simulink model "Resp18e_updatedPulse"  (Simulink 7.3)
settings: Solver=ode23  StartTime=0.0  StopTime=20  FixedStep=0.01  MaxStep=0.05  RelTol=1e-6
values from neighbouring files (symbols this model uses):
  alpha_CO2_brain = 2.9/1e3*760/P_stp/K_stp    (= 0.00097047576489)    [initialize_parameters.m]
  alpha_CO2_fat = 0.9/K_stp/P_stp    (= 0.000396292281489)    [initialize_parameters.m]
  alpha_CO2_heart = 2.4/1e3*760/P_stp/K_stp    (= 0.00080315235715)    [initialize_parameters.m]
  alpha_CO2_lean = 4.2/1e3*760/P_stp/K_stp    (= 0.00140551662501)    [initialize_parameters.m]
  alpha_CO2_lungtiss_fast = alpha_CO2_lungtiss_fast./0.1333    [initialize_parameters.m]
  alpha_CO2_muscle = 4.2/1e3*760/P_stp/K_stp    (= 0.00140551662501)    [initialize_parameters.m]
  alpha_CO2_other = 3.0/1e3*760/P_stp/K_stp    (= 0.00100394044644)    [initialize_parameters.m]
  alpha_O2_fat = 5*0.024/K_stp/P_stp    (= 5.28389708651e-05)    [initialize_parameters.m]
  alpha_O2_tissue = 0.024/K_stp/P_stp    (= 1.0567794173e-05)    [initialize_parameters.m]
  BOHRF0 = O2_SHIFT - T_BLOOD_M_37 * (0.024 + BOHRF * 0.0147) - BOHRF1 * 7.4    (= -3.552)    [initialize_parameters.m]
  BOHRF1 = BOHRF * (1 - T_BLOOD_M_37 * 0.0065)    (= 0.48)    [initialize_parameters.m]
  C_a_CO2_i = 20.8e-3    (= 0.0208)    [initialize_parameters.m]    (also in resp18e_ic_norm.mat = 0.0202734801806)
  C_a_O2_i = 8.95e-3    (= 0.00895)    [initialize_parameters.m]    (also in resp18e_ic_norm.mat = 0.00918087581167)
  CAP_O2 = 0.01 * CAP_O2    (= 0.201)    [initialize_parameters.m]
  Cardiac_duty_cycle = 40    [initialize_parameters.m]
  Co_CO2_brain = 401*K_Co_CO2/1e3/K_stp    (= 0.0107345869894)    [initialize_parameters.m]
  Co_CO2_heart = 487*K_Co_CO2/1e3/K_stp    (= 0.0130367677403)    [initialize_parameters.m]
  Co_CO2_lean = 342*K_Co_CO2/1e3/K_stp    (= 0.00915518391618)    [initialize_parameters.m]
  Co_CO2_muscle = 342*K_Co_CO2/1e3/K_stp    (= 0.00915518391618)    [initialize_parameters.m]
  Co_CO2_other = 355*K_Co_CO2/1e3/K_stp    (= 0.00950318798317)    [initialize_parameters.m]
  DH2ODS = DH2ODS + 0.007 * HB_MEQ * (HB_MEQ - 9) / (13.5 * (13.5 - 9))    (= 0.00498709726946)    [initialize_parameters.m]
  F_insp_alv_alvds = F_v_alv_deadspace / F_insp_hivq    (= 0.00299401197605)    [initialize_parameters.m]
  F_insp_alv_hivq = F_v_alv_hivq      / F_insp_hivq    (= 0.997005988024)    [initialize_parameters.m]
  F_insp_alv_lovq = F_v_alv_lovq      / F_insp_lovq    (= 0.5)    [initialize_parameters.m]
  F_insp_alv_midvq = F_v_alv_midvq     / F_insp_lovq    (= 0.5)    [initialize_parameters.m]
  F_insp_hivq = F_v_alv_deadspace + F_v_alv_hivq    (= 0.334)    [initialize_parameters.m]
  F_insp_lovq = F_v_alv_midvq     + F_v_alv_lovq    (= 0.666)    [initialize_parameters.m]
  Fi_CO2_param_est = 0.01    [initialize_parameters.m]
  Fi_error = 1e-6    (= 1e-06)    [initialize_parameters.m]
  Fi_N2_mean = 1-(Fi_O2_mean + Fi_N2O_mean)    (= 0.65)    [initialize_parameters.m]
  Fi_O2_mean = 0.35    [initialize_parameters.m]
  Fi_O2_param_est = 0.01    [initialize_parameters.m]
  Fq_brain = 0.114    [initialize_parameters.m]
  Fq_error = 1e-8    (= 1e-08)    [initialize_parameters.m]
  Fq_fat = 0.103    [initialize_parameters.m]
  Fq_heart = 0.041    [initialize_parameters.m]
  Fq_hepatic = 0.069    [initialize_parameters.m]
  Fq_kidneys = 0.215    [initialize_parameters.m]
  Fq_lean = 0.090    (= 0.09)    [initialize_parameters.m]
  Fq_lungs_anatomicalshunt = 0.01    [initialize_parameters.m]
  Fq_lungs_hivq = (1-Fq_lungs_pulmshunt-Fq_lungs_anatomicalshunt)    *F_v_alv_hivq/(F_v_alv_hivq+F_v_alv_midvq+F_v_alv_lovq)    (= 0.3)    [initialize_parameters.m]
  Fq_lungs_lovq = (1-Fq_lungs_pulmshunt-Fq_lungs_anatomicalshunt)    *F_v_alv_lovq/(F_v_alv_hivq+F_v_alv_midvq+F_v_alv_lovq)    (= 0.3)    [initialize_parameters.m]
  Fq_lungs_midvq = (1-Fq_lungs_pulmshunt-Fq_lungs_anatomicalshunt)    *F_v_alv_midvq/(F_v_alv_hivq+F_v_alv_midvq+F_v_alv_lovq)    (= 0.3)    [initialize_parameters.m]
  Fq_lungs_pulmshunt = 0.09    [initialize_parameters.m]
  Fq_muscle = 0.096    [initialize_parameters.m]
  Fq_pershunt = 0.101    [initialize_parameters.m]
  Fq_portal = 0.171    [initialize_parameters.m]
  FRC = 2.2    [initialize_parameters.m]
  H2OB = H2OVC + 0.938 * (1 - VC_74)    (= 0.840191964286)    [initialize_parameters.m]
  k_CO2_lungtiss_fast_alvds = k_CO2_lungtiss_fast*F_v_alv_deadspace    (= 3.63090772693e-07)    [initialize_parameters.m]
  k_CO2_lungtiss_fast_hivq = k_CO2_lungtiss_fast*F_v_alv_hivq    (= 0.000120909227307)    [initialize_parameters.m]
  k_CO2_lungtiss_fast_lovq = k_CO2_lungtiss_fast*F_v_alv_lovq    (= 0.000120909227307)    [initialize_parameters.m]
  k_CO2_lungtiss_fast_midvq = k_CO2_lungtiss_fast*F_v_alv_midvq    (= 0.000120909227307)    [initialize_parameters.m]
  k_CO2_lungtiss_slow_alvds = k_CO2_lungtiss_slow*F_v_alv_deadspace    (= 4.95123780945e-09)    [initialize_parameters.m]
  k_CO2_lungtiss_slow_hivq = k_CO2_lungtiss_slow*F_v_alv_hivq    (= 1.64876219055e-06)    [initialize_parameters.m]
  k_CO2_lungtiss_slow_lovq = k_CO2_lungtiss_slow*F_v_alv_lovq    (= 1.64876219055e-06)    [initialize_parameters.m]
  k_CO2_lungtiss_slow_midvq = k_CO2_lungtiss_slow*F_v_alv_midvq    (= 1.64876219055e-06)    [initialize_parameters.m]
  K_diff_CO2_hivq = K_diff_CO2*F_v_alv_hivq    (= 0.0014985)    [initialize_parameters.m]
  K_diff_CO2_lovq = K_diff_CO2*F_v_alv_lovq    (= 0.0014985)    [initialize_parameters.m]
  K_diff_CO2_midvq = K_diff_CO2*F_v_alv_midvq    (= 0.0014985)    [initialize_parameters.m]
  K_diff_O2_hivq = K_diff_O2*F_v_alv_hivq    (= 7.326e-05)    [initialize_parameters.m]
  K_diff_O2_lovq = K_diff_O2*F_v_alv_lovq    (= 7.326e-05)    [initialize_parameters.m]
  K_diff_O2_midvq = K_diff_O2*F_v_alv_midvq    (= 7.326e-05)    [initialize_parameters.m]
  K_exp_alv_alvds = 1/1    (= 1)    [initialize_parameters.m]
  K_exp_alv_hivq = 1/1    (= 1)    [initialize_parameters.m]
  K_press = 760/101.325    (= 7.50061682704)    [initialize_parameters.m]
  K_stp = R*(T_stp+273.15)/(P_stp*1000)    (= 22.4135311621)    [initialize_parameters.m]
  Kg_alv = R*(T_alv+273.15)/(P_baro*1000)    (= 25.3668469802)    [initialize_parameters.m]
  LN10 = 2.30258509299405    (= 2.30258509299)    [initialize_parameters.m]
  m_alv_alvds_i = (FRC-V_deadspace_total)/Kg_alv * F_v_alv_deadspace    [initialize_parameters.m]
  m_alv_hivq_i = (FRC-V_deadspace_total)/Kg_alv * F_v_alv_hivq    [initialize_parameters.m]
  m_alv_lovq_i = (FRC-V_deadspace_total)/Kg_alv * F_v_alv_lovq    [initialize_parameters.m]
  m_alv_midvq_i = (FRC-V_deadspace_total)/Kg_alv * F_v_alv_midvq    [initialize_parameters.m]
  m_CO2_alv_alvds_i = F_CO2_i * m_alv_alvds_i    [initialize_parameters.m]
  m_CO2_alv_hivq_i = F_CO2_i * m_alv_hivq_i    [initialize_parameters.m]
  m_CO2_alv_lovq_i = F_CO2_i * m_alv_lovq_i    [initialize_parameters.m]
  m_CO2_alv_midvq_i = F_CO2_i * m_alv_midvq_i    [initialize_parameters.m]
  m_CO2_brain_b_i = C_a_CO2_i*Vb_brain    (= 0.002184)    [initialize_parameters.m]
  m_CO2_brain_t_i = (Co_CO2_brain  + alpha_CO2_brain *P_v_CO2_i)* Vt_brain    (= 0.0171268217946)    [initialize_parameters.m]
  m_CO2_common_b_i = C_a_CO2_i*Vb_common    (= 0.0170421333333)    [initialize_parameters.m]
  m_CO2_ds0_i = F_CO2_i*m_ds0_i    (= 0.000985538329597)    [initialize_parameters.m]
  m_CO2_ds_large_i = F_CO2_i * m_deadspace_large_1    [initialize_parameters.m]
  m_CO2_ds_med_hivq1_i = F_CO2_i * m_deadspace_med_hivq_1    [initialize_parameters.m]
  m_CO2_ds_med_hivq2_i = F_CO2_i * m_deadspace_med_hivq_2    [initialize_parameters.m]
  m_CO2_ds_med_lovq1_i = F_CO2_i * m_deadspace_med_lovq_1    [initialize_parameters.m]
  m_CO2_ds_med_lovq2_i = F_CO2_i * m_deadspace_med_lovq_2    [initialize_parameters.m]
  m_CO2_ds_small_alvds_i = F_CO2_i * m_deadspace_small_alvdeadspace    [initialize_parameters.m]
  m_CO2_ds_small_hivq_i = F_CO2_i * m_deadspace_small_hivq    [initialize_parameters.m]
  m_CO2_ds_small_lovq_i = F_CO2_i * m_deadspace_small_lovq    [initialize_parameters.m]
  m_CO2_ds_small_midvq_i = F_CO2_i * m_deadspace_small_midvq    [initialize_parameters.m]
  m_CO2_fat_b_i = C_a_CO2_i*Vb_fat    (= 0.0116896)    [initialize_parameters.m]
  m_CO2_fat_t_i = P_a_CO2_i*alpha_CO2_fat*Vt_fat    (= 0.0302752719501)    [initialize_parameters.m]
  m_CO2_heart_b_i = C_a_CO2_i*Vb_heart    (= 0.000832)    [initialize_parameters.m]
  m_CO2_heart_t_i = (Co_CO2_heart  + alpha_CO2_heart *P_v_CO2_i)* Vt_heart    (= 0.00402544335149)    [initialize_parameters.m]
  m_CO2_hepatic_b_i = C_a_CO2_i*Vb_hepatic    (= 0.0019136)    [initialize_parameters.m]
  m_CO2_kidneys_b_i = C_a_CO2_i*Vb_kidneys    (= 0.0012064)    [initialize_parameters.m]
  m_CO2_kidneys_t_i = (Co_CO2_other  + alpha_CO2_other *P_v_CO2_i)* Vt_kidneys    (= 0.0045902552907)    [initialize_parameters.m]
  m_CO2_lean_b_i = C_a_CO2_i*Vb_lean    (= 0.0191984)    [initialize_parameters.m]
  m_CO2_lean_t_i = (Co_CO2_lean   + alpha_CO2_lean  *P_v_CO2_i)* Vt_lean    (= 0.0884995401953)    [initialize_parameters.m]
  m_CO2_liver_t_i = (Co_CO2_other  + alpha_CO2_other *P_v_CO2_i)* Vt_liver    (= 0.0187019339777)    [initialize_parameters.m]
  m_CO2_lungtiss_fast_alvds_i = F_CO2_i*(P_baro-P_A_H2O)*V_lungtiss_alvds *alpha_CO2_lungtiss_fast(2)    [initialize_parameters.m]
  m_CO2_lungtiss_fast_hivq_i = F_CO2_i*(P_baro-P_A_H2O)*V_lungtiss_hivq  *alpha_CO2_lungtiss_fast(2)    [initialize_parameters.m]
  m_CO2_lungtiss_fast_lovq_i = F_CO2_i*(P_baro-P_A_H2O)*V_lungtiss_lovq  *alpha_CO2_lungtiss_fast(2)    [initialize_parameters.m]
  m_CO2_lungtiss_fast_midvq_i = F_CO2_i*(P_baro-P_A_H2O)*V_lungtiss_midvq *alpha_CO2_lungtiss_fast(2)    [initialize_parameters.m]
  m_CO2_lungtiss_slow_alvds_i = F_CO2_i*(P_baro-P_A_H2O)*V_lungtiss_alvds*alpha_CO2_lungtiss_slow    [initialize_parameters.m]
  m_CO2_lungtiss_slow_hivq_i = F_CO2_i*(P_baro-P_A_H2O)*V_lungtiss_hivq *alpha_CO2_lungtiss_slow    [initialize_parameters.m]
  m_CO2_lungtiss_slow_lovq_i = F_CO2_i*(P_baro-P_A_H2O)*V_lungtiss_lovq *alpha_CO2_lungtiss_slow    [initialize_parameters.m]
  m_CO2_lungtiss_slow_midvq_i = F_CO2_i*(P_baro-P_A_H2O)*V_lungtiss_midvq*alpha_CO2_lungtiss_slow    [initialize_parameters.m]
  m_CO2_LV_b_i = C_a_CO2_i*Vb_LV    (= 0.00391733333333)    [initialize_parameters.m]
  m_CO2_muscle_b_i = C_a_CO2_i*Vb_muscle    (= 0.0201344)    [initialize_parameters.m]
  m_CO2_muscle_t_i = (Co_CO2_muscle + alpha_CO2_muscle*P_v_CO2_i)* Vt_muscle    (= 0.363660431061)    [initialize_parameters.m]
  m_CO2_pershunt_b_i = C_a_CO2_i*Vb_pershunt    (= 0.0027248)    [initialize_parameters.m]
  m_CO2_portal_b_i = C_a_CO2_i*Vb_portal    (= 0.0210912)    [initialize_parameters.m]
  m_CO2_portal_t_i = (Co_CO2_other  + alpha_CO2_other *P_v_CO2_i)* Vt_portal    (= 0.0164739329706)    [initialize_parameters.m]
  m_CO2_pulmcap_b_hivq_i = C_a_CO2_i*Vb_pulmcap_hivq    (= 0.000630933333333)    [initialize_parameters.m]
  m_CO2_pulmcap_b_lovq_i = C_a_CO2_i*Vb_pulmcap_lovq    (= 0.000630933333333)    [initialize_parameters.m]
  m_CO2_pulmcap_b_midvq_i = C_a_CO2_i*Vb_pulmcap_midvq    (= 0.000630933333333)    [initialize_parameters.m]
  m_CO2_pulmcap_b_pulmshunt_i = C_a_CO2_i*Vb_pulmcap_pulmshunt    (= 0.0001872)    [initialize_parameters.m]
  m_CO2_RV_b_i = C_v_CO2_i*Vb_RV    (= 0.004181)    [initialize_parameters.m]
  m_N2_alv_alvds_i = Fi_N2_mean * (m_alv_alvds_i - m_CO2_alv_alvds_i)    [initialize_parameters.m]
  ... (+122 more)
undefined symbols (not defined in the file or in its folder): AH2OVC, AHCO3B, DHCO3BDS, litres, mole
libraries: simulink x28
(part 2 of 8)

== system Resp18e_updatedPulse/Patient/Pulm cap Hi V/Q ==
  note: This block calculates:
      | 1. Alveolar partial pressures of CO2 & O2
      | 2. CO2 uptake by lung tissues
      | 3. CO2 uptake by pulmonary capillaries
      | 4. O2 uptake by pulmonary capillaries
  note: Variables:
      | CA_CO2: alveolar CO2 fraction (pu)
      | CA_O2: alveolar O2 fraction (pu)
      | P_baro: barometric pressure (kPa)
      | P_alv: gauge pressure in alveolar compartment (kPa)
      | P_H2O_alv: partial press of H2O vapour in alveolar compartment (kPa)
      | C_v_CO2: mixed venous CO2 concentration (moles/l)
      | C_v_O2: mixed venous O2 concentration (moles/l)
      | Qpdot: pulmonary blood flow (l/sec)
      | mdot_CO2_tiss_cap: flux of CO2 from alv to tissues + pulm capillaries (mole/sec)
      | mdot_O2_tiss_cap: flux of O2 from alv to tissues + pulm capillaries (mole/sec)
      | Cec_CO2 CO2 conc at end of pulm capillaries
      | Cec_O2 O2 conc at end of pulm capillaries
      | CaCO2: arterial CO2 concentration (moles/l)
      | CaO2: arterial O2 concentration (moles/l)
  FA_gases : Inport  PortDimensions=2  OutDataType=sfix(16)  OutScaling=2^0
  C_v_gases : Inport  Port=2  PortDimensions=2  OutDataType=sfix(16)  OutScaling=2^0
  CO2 O2 : Mux  Inputs=2
  Demux : Demux  Outputs=2
  Lung tissue : Subsystem  Description=Calculates quantity of CO2 stored in two lung tissue compartments (fast & slow)
  Net inflow CO4 : Sum  OutDataType=sfix(16)  OutScaling=2^0  SaturateOnIntegerOverflow=on  InputSameDT=on  OutDataTypeStr=Inherit: Same as first input
  P3 : Product  Inputs=**  OutDataType=sfix(16)  OutScaling=2^0  SaturateOnIntegerOverflow=on  RndMeth=Zero  InputSameDT=on  OutDataTypeStr=Inherit: Same as first input
  P4 : Product  Inputs=**  OutDataType=sfix(16)  OutScaling=2^0  SaturateOnIntegerOverflow=on  RndMeth=Zero  InputSameDT=on  OutDataTypeStr=Inherit: Same as first input
  Pulm capillaries : Subsystem
  To Workspace16 : ToWorkspace  VariableName=mdot_CO2_a_A_hivq  SampleTime=t_sample  SaveFormat=Array
  To Workspace8 : ToWorkspace  VariableName=P_A_CO2_hivq  SampleTime=t_sample  SaveFormat=Array
  To Workspace9 : ToWorkspace  VariableName=P_A_O2_hivq  SampleTime=t_sample  SaveFormat=Array
  sum3 : Sum  Inputs=++-  OutDataType=sfix(16)  OutScaling=2^0  SaturateOnIntegerOverflow=on  InputSameDT=on  OutDataTypeStr=Inherit: Same as first input
  mdot_gases : Outport  OutDataType=sfix(16)  OutScaling=2^0
  C_gases : Outport  Port=2  OutDataType=sfix(16)  OutScaling=2^0
  tag scope: mdot_CO2_a_A_hivq=global, mdot_O2_a_A_hivq=global
  wires:
  Lung tissue/1(mdot_CO2_tissue) -> Net inflow CO4/1
  sum3/1 -> P3/2, P4/2
  P3/1 -> Pulm capillaries/1(PA_CO2), Lung tissue/1(PA_CO2), To Workspace8/1  "PA_CO2"
  Demux/2 -> P4/1
  P4/1 -> Pulm capillaries/2(PA_O2), To Workspace9/1  "PA_O2"
  Demux/1 -> P3/1
  Net inflow CO4/1 -> CO2 O2/1
  CO2 O2/1 -> mdot_gases/1
  [P_alv] -> sum3/2
  FA_gases/1 -> Demux/1
  Pulm capillaries/1(mdot_CO2_A_a) -> Net inflow CO4/2, To Workspace16/1, [mdot_CO2_a_A_hivq]
  [P_A_H2O] -> sum3/3
  [P_baro] -> sum3/1
  C_v_gases/1 -> Pulm capillaries/3(C_v_gases)
  Pulm capillaries/3(Cec_gases) -> C_gases/1
  Pulm capillaries/2(mdot_O2_A_a) -> CO2 O2/2, [mdot_O2_a_A_hivq]

== system Resp18e_updatedPulse/Patient/Pulm cap Lo V/Q ==
  note: This block calculates:
      | 1. Alveolar partial pressures of CO2 & O2
      | 2. CO2 uptake by lung tissues
      | 3. CO2 uptake by pulmonary capillaries
      | 4. O2 uptake by pulmonary capillaries
  note: Variables:
      | CA_CO2: alveolar CO2 fraction (pu)
      | CA_O2: alveolar O2 fraction (pu)
      | P_baro: barometric pressure (kPa)
      | P_alv: gauge pressure in alveolar compartment (kPa)
      | P_H2O_alv: partial press of H2O vapour in alveolar compartment (kPa)
      | C_v_CO2: mixed venous CO2 concentration (moles/l)
      | C_v_O2: mixed venous O2 concentration (moles/l)
      | Qpdot: pulmonary blood flow (l/sec)
      | mdot_CO2_tiss_cap: flux of CO2 from alv to tissues + pulm capillaries (mole/sec)
      | mdot_O2_tiss_cap: flux of O2 from alv to tissues + pulm capillaries (mole/sec)
      | Cec_CO2 CO2 conc at end of pulm capillaries
      | Cec_O2 O2 conc at end of pulm capillaries
      | CaCO2: arterial CO2 concentration (moles/l)
      | CaO2: arterial O2 concentration (moles/l)
  FA_gases : Inport  PortDimensions=2  OutDataType=sfix(16)  OutScaling=2^0
  C_v_gases : Inport  Port=2  PortDimensions=2  OutDataType=sfix(16)  OutScaling=2^0
  CO2 O2 : Mux  Inputs=2
  Demux : Demux  Outputs=2
  Lung tissue : Subsystem  Description=Calculates quantity of CO2 stored in two lung tissue compartments (fast & slow)
  Net inflow CO4 : Sum  OutDataType=sfix(16)  OutScaling=2^0  SaturateOnIntegerOverflow=on  InputSameDT=on  OutDataTypeStr=Inherit: Same as first input
  P3 : Product  Inputs=**  OutDataType=sfix(16)  OutScaling=2^0  SaturateOnIntegerOverflow=on  RndMeth=Zero  InputSameDT=on  OutDataTypeStr=Inherit: Same as first input
  P4 : Product  Inputs=**  OutDataType=sfix(16)  OutScaling=2^0  SaturateOnIntegerOverflow=on  RndMeth=Zero  InputSameDT=on  OutDataTypeStr=Inherit: Same as first input
  Pulm capillaries : Subsystem
  To Workspace16 : ToWorkspace  VariableName=mdot_CO2_a_A_lovq  SampleTime=t_sample  SaveFormat=Array
  To Workspace8 : ToWorkspace  VariableName=P_A_CO2_lovq  SampleTime=t_sample  SaveFormat=Array
  To Workspace9 : ToWorkspace  VariableName=P_A_O2_lovq  SampleTime=t_sample  SaveFormat=Array
  sum3 : Sum  Inputs=++-  OutDataType=sfix(16)  OutScaling=2^0  SaturateOnIntegerOverflow=on  InputSameDT=on  OutDataTypeStr=Inherit: Same as first input
  mdot_gases : Outport  OutDataType=sfix(16)  OutScaling=2^0
  C_gases : Outport  Port=2  OutDataType=sfix(16)  OutScaling=2^0
  tag scope: mdot_CO2_a_A_lovq=global, mdot_O2_a_A_lovq=global
  wires:
  Lung tissue/1(mdot_CO2_tissue) -> Net inflow CO4/1
  sum3/1 -> P3/2, P4/2
  P3/1 -> Pulm capillaries/1(PA_CO2), Lung tissue/1(PA_CO2), To Workspace8/1  "PA_CO2"
  Demux/2 -> P4/1
  P4/1 -> Pulm capillaries/2(PA_O2), To Workspace9/1  "PA_O2"
  Demux/1 -> P3/1
  Net inflow CO4/1 -> CO2 O2/1
  CO2 O2/1 -> mdot_gases/1
  [P_alv] -> sum3/2
  FA_gases/1 -> Demux/1
  Pulm capillaries/1(mdot_CO2_A_a) -> Net inflow CO4/2, To Workspace16/1, [mdot_CO2_a_A_lovq]
  [P_A_H2O] -> sum3/3
  [P_baro] -> sum3/1
  C_v_gases/1 -> Pulm capillaries/3(C_v_gases)
  Pulm capillaries/3(Cec_gases) -> C_gases/1
  Pulm capillaries/2(mdot_O2_A_a) -> CO2 O2/2, [mdot_O2_a_A_lovq]

== system Resp18e_updatedPulse/Patient/Pulm cap Mid V/Q ==
  note: Variables:
      | CA_CO2: alveolar CO2 fraction (pu)
      | CA_O2: alveolar O2 fraction (pu)
      | P_baro: barometric pressure (kPa)
      | P_alv: gauge pressure in alveolar compartment (kPa)
      | P_H2O_alv: partial press of H2O vapour in alveolar compartment (kPa)
      | C_v_CO2: mixed venous CO2 concentration (moles/l)
      | C_v_O2: mixed venous O2 concentration (moles/l)
      | Qpdot: pulmonary blood flow (l/sec)
      | mdot_CO2_tiss_cap: flux of CO2 from alv to tissues + pulm capillaries (mole/sec)
      | mdot_O2_tiss_cap: flux of O2 from alv to tissues + pulm capillaries (mole/sec)
      | Cec_CO2 CO2 conc at end of pulm capillaries
      | Cec_O2 O2 conc at end of pulm capillaries
      | CaCO2: arterial CO2 concentration (moles/l)
      | CaO2: arterial O2 concentration (moles/l)
  note: This block calculates:
      | 1. Alveolar partial pressures of CO2 & O2
      | 2. CO2 uptake by lung tissues
      | 3. CO2 uptake by pulmonary capillaries
      | 4. O2 uptake by pulmonary capillaries
  FA_gases : Inport  PortDimensions=2  OutDataType=sfix(16)  OutScaling=2^0
  C_v_gases : Inport  Port=2  PortDimensions=2  OutDataType=sfix(16)  OutScaling=2^0
  CO2 O2 : Mux  Inputs=2
  Demux : Demux  Outputs=2
  Lung tissue : Subsystem  Description=Calculates quantity of CO2 stored in two lung tissue compartments (fast & slow)
  Net inflow CO4 : Sum  OutDataType=sfix(16)  OutScaling=2^0  SaturateOnIntegerOverflow=on  InputSameDT=on  OutDataTypeStr=Inherit: Same as first input
  P3 : Product  Inputs=**  OutDataType=sfix(16)  OutScaling=2^0  SaturateOnIntegerOverflow=on  RndMeth=Zero  InputSameDT=on  OutDataTypeStr=Inherit: Same as first input
  P4 : Product  Inputs=**  OutDataType=sfix(16)  OutScaling=2^0  SaturateOnIntegerOverflow=on  RndMeth=Zero  InputSameDT=on  OutDataTypeStr=Inherit: Same as first input
  Pulm capillaries : Subsystem
  To Workspace16 : ToWorkspace  VariableName=mdot_CO2_a_A_midvq  SampleTime=t_sample  SaveFormat=Array
  To Workspace17 : ToWorkspace  VariableName=mdot_CO2_A_midvq  SampleTime=t_sample  SaveFormat=Array
  To Workspace8 : ToWorkspace  VariableName=P_A_CO2_midvq  SampleTime=t_sample  SaveFormat=Array
  To Workspace9 : ToWorkspace  VariableName=P_A_O2_midvq  SampleTime=t_sample  SaveFormat=Array
  sum3 : Sum  Inputs=++-  OutDataType=sfix(16)  OutScaling=2^0  SaturateOnIntegerOverflow=on  InputSameDT=on  OutDataTypeStr=Inherit: Same as first input
  mdot_gases : Outport  OutDataType=sfix(16)  OutScaling=2^0
  C_gases : Outport  Port=2  OutDataType=sfix(16)  OutScaling=2^0
  tag scope: mdot_CO2_a_A_midvq=global, mdot_O2_a_A_midvq=global
  wires:
  Pulm capillaries/3(Cec_gases) -> C_gases/1
  C_v_gases/1 -> Pulm capillaries/3(C_v_gases)
  [P_baro] -> sum3/1
  [P_A_H2O] -> sum3/3
  Pulm capillaries/1(mdot_CO2_A_a) -> Net inflow CO4/2, To Workspace16/1, [mdot_CO2_a_A_midvq]
  FA_gases/1 -> Demux/1
  [P_alv] -> sum3/2
  CO2 O2/1 -> mdot_gases/1
  Demux/1 -> P3/1
  P4/1 -> To Workspace9/1, Pulm capillaries/2(PA_O2)  "PA_O2"
  Demux/2 -> P4/1
  P3/1 -> To Workspace8/1, Lung tissue/1(PA_CO2), Pulm capillaries/1(PA_CO2)  "PA_CO2"
  sum3/1 -> P4/2, P3/2
  Lung tissue/1(mdot_CO2_tissue) -> Net inflow CO4/1
  Net inflow CO4/1 -> CO2 O2/1, To Workspace17/1
  Pulm capillaries/2(mdot_O2_A_a) -> CO2 O2/2, [mdot_O2_a_A_midvq]

== system Resp18e_updatedPulse/Patient/Pulm cap pulm shunt ==
  note: Pulmonary capillary shunt
  note: This block calculates mixing and effective delay in pulmonary capillary compartment that is not exposed to alveolar gas
      | Note that the time constant of this 1st order loop should be approx independent of V_b_pulmcap_pulmshunt if
      | V_b_pulmcap_pulmshunt is approx proportional to Fq_lung_pulmshunt
  C_v_gases : Inport  PortDimensions=2  OutDataType=sfix(16)  OutScaling=2^0
  CO2_cap : Integrator  InitialCondition=m_CO2_pulmcap_b_pulmshunt_i
  C_CO2 body : Gain  Gain=1/Vb_pulmcap_pulmshunt  ParameterDataType=sfix(16)  ParameterScaling=2^0  OutDataType=sfix(16)  OutScaling=2^0  SaturateOnIntegerOverflow=on  OutDataTypeStr=Inherit: Same as input  ParamDataTypeStr=Inherit: Same as input
  C_O2 body : Gain  Gain=1/Vb_pulmcap_pulmshunt  ParameterDataType=sfix(16)  ParameterScaling=2^0  OutDataType=sfix(16)  OutScaling=2^0  SaturateOnIntegerOverflow=on  OutDataTypeStr=Inherit: Same as input  ParamDataTypeStr=Inherit: Same as input
  Demux2 : Demux  Outputs=2
  Mux1 : Mux  Inputs=2
  Net inflow CO5 : Sum  Inputs=+-  OutDataType=sfix(16)  OutScaling=2^0  SaturateOnIntegerOverflow=on  InputSameDT=on  OutDataTypeStr=Inherit: Same as first input
  Net inflow CO6 : Sum  Inputs=+-  OutDataType=sfix(16)  OutScaling=2^0  SaturateOnIntegerOverflow=on  InputSameDT=on  OutDataTypeStr=Inherit: Same as first input
  O2_cap : Integrator  InitialCondition=m_O2_pulmcap_b_pulmshunt_i
  P11 : Product  Inputs=**  OutDataType=sfix(16)  OutScaling=2^0  SaturateOnIntegerOverflow=on  RndMeth=Zero  InputSameDT=on  OutDataTypeStr=Inherit: Same as first input
  P8 : Product  Inputs=**  OutDataType=sfix(16)  OutScaling=2^0  SaturateOnIntegerOverflow=on  RndMeth=Zero  InputSameDT=on  OutDataTypeStr=Inherit: Same as first input
  P9 : Product  Inputs=**  OutDataType=sfix(16)  OutScaling=2^0  SaturateOnIntegerOverflow=on  RndMeth=Zero  InputSameDT=on  OutDataTypeStr=Inherit: Same as first input
  Cec_gases : Outport  OutDataType=sfix(16)  OutScaling=2^0
  wires:
  CO2_cap/1 -> C_CO2 body/1
  O2_cap/1 -> C_O2 body/1
  Net inflow CO5/1 -> P8/1
  Demux2/1 -> Net inflow CO5/1
  Demux2/2 -> Net inflow CO6/1
  Net inflow CO6/1 -> P9/2
  P8/1 -> CO2_cap/1
  P9/1 -> O2_cap/1
  C_CO2 body/1 -> Net inflow CO5/2, Mux1/1
  C_O2 body/1 -> Net inflow CO6/2, Mux1/2
  Mux1/1 -> Cec_gases/1
  [Fq_lungs_pulmshunt] -> P11/2
  P11/1 -> P8/2, P9/1
  C_v_gases/1 -> Demux2/1
  [Qpdot] -> P11/1

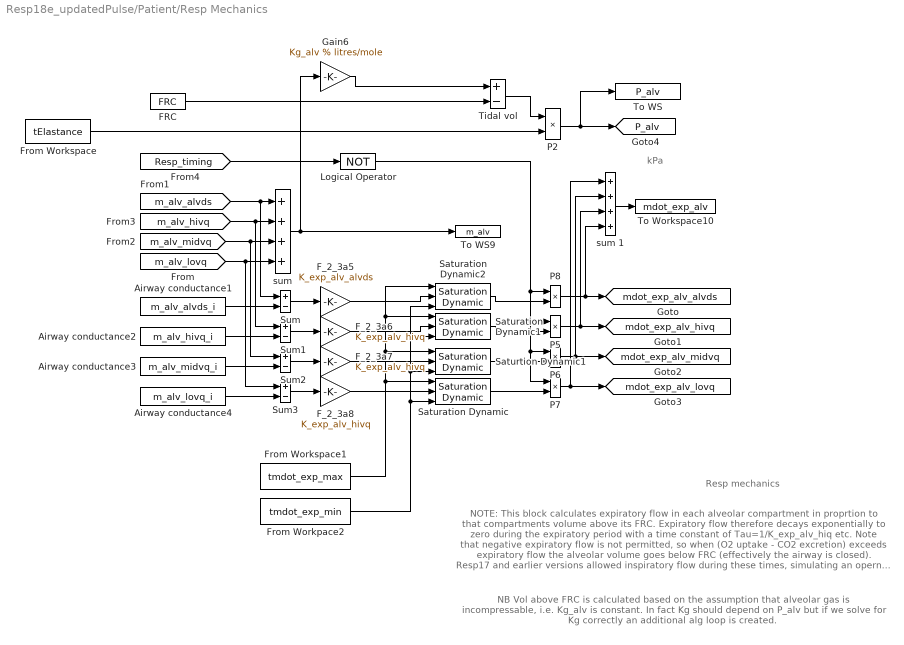
== system Resp18e_updatedPulse/Patient/Resp Mechanics ==
  note: Resp mechanics
  note: NB Vol above FRC is calculated based on the assumption that alveolar gas is incompressable, i.e. Kg_alv
      | is constant. In fact Kg should depend on P_alv but if we solve for Kg correctly an additional alg loop is created.
  note: kPa
  note: NOTE: This block calculates expiratory flow in each alveolar compartment in proprtion to that
      | compartments volume above its FRC. Expiratory flow therefore decays exponentially to
      | zero during the expiratory period with a time constant of Tau=1/K_exp_alv_hiq etc.
      | Note that negative expiratory flow is not permitted, so when (O2 uptake - CO2 excretion)
      | exceeds expiratory flow the alveolar volume goes below FRC (effectively the airway is closed).
      | Resp17 and earlier versions allowed inspiratory flow during these times, simulating an opern airway.
  Airway conductance1 : Constant  Value=m_alv_alvds_i  OutDataType=sfix(16)  OutScaling=2^0
  Airway conductance2 : Constant  Value=m_alv_hivq_i  OutDataType=sfix(16)  OutScaling=2^0
  Airway conductance3 : Constant  Value=m_alv_midvq_i  OutDataType=sfix(16)  OutScaling=2^0
  Airway conductance4 : Constant  Value=m_alv_lovq_i  OutDataType=sfix(16)  OutScaling=2^0
  FRC : Constant  Value=FRC  OutDataType=sfix(16)  OutScaling=2^0
  F_2_3a5 : Gain  Gain=K_exp_alv_alvds  ParameterDataType=sfix(16)  ParameterScaling=2^0  OutDataType=sfix(16)  OutScaling=2^0  SaturateOnIntegerOverflow=on  OutDataTypeStr=Inherit: Same as input  ParamDataTypeStr=Inherit: Same as input
  F_2_3a6 : Gain  Gain=K_exp_alv_hivq  ParameterDataType=sfix(16)  ParameterScaling=2^0  OutDataType=sfix(16)  OutScaling=2^0  SaturateOnIntegerOverflow=on  OutDataTypeStr=Inherit: Same as input  ParamDataTypeStr=Inherit: Same as input
  F_2_3a7 : Gain  Gain=K_exp_alv_hivq  ParameterDataType=sfix(16)  ParameterScaling=2^0  OutDataType=sfix(16)  OutScaling=2^0  SaturateOnIntegerOverflow=on  OutDataTypeStr=Inherit: Same as input  ParamDataTypeStr=Inherit: Same as input
  F_2_3a8 : Gain  Gain=K_exp_alv_hivq  ParameterDataType=sfix(16)  ParameterScaling=2^0  OutDataType=sfix(16)  OutScaling=2^0  SaturateOnIntegerOverflow=on  OutDataTypeStr=Inherit: Same as input  ParamDataTypeStr=Inherit: Same as input
  From Workpace2 : FromWorkspace  VariableName=tmdot_exp_min  SampleTime=0  Interpolate=off  OutputAfterFinalValue=Holding final value
  From Workspace : FromWorkspace  VariableName=tElastance  SampleTime=0  Interpolate=off  OutputAfterFinalValue=Holding final value
  From Workspace1 : FromWorkspace  VariableName=tmdot_exp_max  SampleTime=0  Interpolate=off  OutputAfterFinalValue=Holding final value
  Gain6 : Gain  Gain=Kg_alv % litres/mole  ParameterDataType=sfix(16)  ParameterScaling=2^0  OutDataType=sfix(16)  OutScaling=2^0  SaturateOnIntegerOverflow=on  OutDataTypeStr=Inherit: Same as input  ParamDataTypeStr=Inherit: Same as input
  Logical Operator : Logic  Operator=NOT
  P{2,5..8} (5 alike) : Product  OutDataType=sfix(16)  OutScaling=2^0  SaturateOnIntegerOverflow=on  RndMeth=Zero  InputSameDT=on  OutDataTypeStr=Inherit: Same as first input
  Saturation Dynamic : simulink/Discontinuities/Saturation Dynamic  SystemSampleTime=-1  OutMin=[]  OutMax=[]  OutDataTypeStr=Inherit: Same as second input  OutDataType=fixdt(1, 16)  OutScaling=2^-10  DoSatur=off
  Saturation Dynamic1 : simulink/Discontinuities/Saturation Dynamic  SystemSampleTime=-1  OutMin=[]  OutMax=[]  OutDataTypeStr=Inherit: Same as second input  OutDataType=fixdt(1, 16)  OutScaling=2^-10  DoSatur=off
  Saturation Dynamic2 : simulink/Discontinuities/Saturation Dynamic  SystemSampleTime=-1  OutMin=[]  OutMax=[]  OutDataTypeStr=Inherit: Same as second input  OutDataType=fixdt(1, 16)  OutScaling=2^-10  DoSatur=off
  Saturtion Dynamic1 : simulink/Discontinuities/Saturation Dynamic  SystemSampleTime=-1  OutMin=[]  OutMax=[]  OutDataTypeStr=Inherit: Same as second input  OutDataType=fixdt(1, 16)  OutScaling=2^-10  DoSatur=off
  Sum{,1..3} (4 alike) : Sum  Inputs=+-  OutDataType=sfix(16)  OutScaling=2^0  SaturateOnIntegerOverflow=on  InputSameDT=on  OutDataTypeStr=Inherit: Same as first input
  Tidal vol : Sum  Inputs=+-  OutDataType=sfix(16)  OutScaling=2^0  SaturateOnIntegerOverflow=on  InputSameDT=on  OutDataTypeStr=Inherit: Same as first input
  To WS : ToWorkspace  VariableName=P_alv  SampleTime=t_sample  SaveFormat=Array
  To WS9 : ToWorkspace  VariableName=m_alv  SampleTime=t_sample  SaveFormat=Array
  To Workspace10 : ToWorkspace  VariableName=mdot_exp_alv  SampleTime=t_sample  SaveFormat=Array
  "sum " : Sum  Inputs=++++  OutDataType=sfix(16)  OutScaling=2^0  SaturateOnIntegerOverflow=on  InputSameDT=on  OutDataTypeStr=Inherit: Same as first input
  sum 1 : Sum  Inputs=++++  OutDataType=sfix(16)  OutScaling=2^0  SaturateOnIntegerOverflow=on  InputSameDT=on  OutDataTypeStr=Inherit: Same as first input
  tag scope: P_alv=global, mdot_exp_alv_alvds=global, mdot_exp_alv_hivq=global, mdot_exp_alv_lovq=global, mdot_exp_alv_midvq=global
  wires:
  [m_alv_alvds] -> "sum "/1, Sum/1
  Airway conductance1/1 -> Sum/2
  Airway conductance2/1 -> Sum1/2
  Airway conductance3/1 -> Sum2/2
  Airway conductance4/1 -> Sum3/2
  [m_alv_hivq] -> "sum "/2, Sum1/1
  [m_alv_midvq] -> "sum "/3, Sum2/1
  [m_alv_lovq] -> "sum "/4, Sum3/1
  Sum/1 -> F_2_3a5/1
  F_2_3a5/1 -> Saturation Dynamic2/2
  F_2_3a6/1 -> Saturation Dynamic1/2
  Sum1/1 -> F_2_3a6/1
  F_2_3a7/1 -> Saturtion Dynamic1/2
  F_2_3a8/1 -> Saturation Dynamic/2
  Sum2/1 -> F_2_3a7/1
  Sum3/1 -> F_2_3a8/1
  Saturation Dynamic2/1 -> P8/2
  Saturation Dynamic1/1 -> P5/2
  Saturation Dynamic/1 -> P7/2
  Saturtion Dynamic1/1 -> P6/2
  Logical Operator/1 -> P8/1, P5/1, P6/1, P7/1
  FRC/1 -> Tidal vol/2
  Tidal vol/1 -> P2/1
  Gain6/1 -> Tidal vol/1
  From Workspace/1 -> P2/2
  "sum "/1 -> To WS9/1, Gain6/1
  P2/1 -> To WS/1, [P_alv]
  sum 1/1 -> To Workspace10/1
  P8/1 -> [mdot_exp_alv_alvds], sum 1/4
  P5/1 -> [mdot_exp_alv_hivq], sum 1/3
  P6/1 -> [mdot_exp_alv_midvq], sum 1/2
  P7/1 -> [mdot_exp_alv_lovq], sum 1/1
  [Resp_timing] -> Logical Operator/1
  From Workspace1/1 -> Saturation Dynamic2/1, Saturation Dynamic1/1, Saturtion Dynamic1/1, Saturation Dynamic/1
  From Workpace2/1 -> Saturation Dynamic2/3, Saturation Dynamic1/3, Saturtion Dynamic1/3, Saturation Dynamic/3

== system Resp18e_updatedPulse/Patient/Resp18e Info ==
  note: Initial conditions and parameters taken from work space
  note: Grodins 5 contains an arterial conmpartment, and Simulink variable delays.
  note: Uses Grodins tissue dissociation curves
  note: Grodins5a has Pulm capillary blood compartment
  note: Grodins6 has body tissue compartment
  note: Grodins 7 closes the loop - feeds body venous blood back to mixed venous input
  note: Grodins8 has a 1st order component simulating mixing in heart & aorta
  note: Grodins10 has multiple body compartments
  note: Grodins11 has xport delays in pulmonary artery & vein, & shunt around pulm capillaries
  note: Grodins12 has more than 2 body compartments
  note: Pulm vein + pulm art delays lumped into one
  note: Grodins13 has multiple body compartments based on Mapleson's models
  note: Grodins14 for trying out rebreathing & sinusoid measurements
  note: Grodins15 has high pass filter in CO2 delivery signal to try to cancel the lung ventilation pole
  note: Resp15 has linear tissue CO2 dissociation curves with values from Fahri & Rahn 1960
  note: Resp 16 uses Olszowka's diss curves
  note: Resp 17 has four lung compartments each with their own perfusion. Pure shunt remains
  note: All lung parameters (tissue vol, ventilation diffusion coeffts) etc are set proportional to compartment volumes
  note: Resp18 created to change expiratory flow calculations so that each alv compartment has exp flow in proportion
      | to its volume Exp flow calculated for each alv compartment separately using a time constant parameter
  note: Resp18a has additional integrators for measuring expired CO2 per breath
      | and code for delivering inspired m_CO2 equal to expired m_CO2
  note: Resp18b has code for delivering sinusoidal inspired CO2
  note: Resp18c: identical to Resp18b but has arterial O2 saturation monitoring
  note: Resp18d has pulse generator to control rebreathing so rebreathing measurements can be repeated
  note: Resp18e can deliver CO2 & O2 pulses and decreases inspired N2 accordingly. Developed
      | to generate 'measured' data from which alveolar vol, dead space, mixed venous CO2
      | & O2 and PBF parameter estimation can be done.

== system Resp18e_updatedPulse/Patient/Airways + alveoli/Alv compartment alvds ==
  note: molar conc
      | per unit
  note: +ve out of alv
  Insp flow in : Inport  PortDimensions=4  OutDataType=sfix(16)  OutScaling=2^0
  mdot_gases : Inport  Port=2  PortDimensions=2  OutDataType=sfix(16)  OutScaling=2^0
  Alv vol : Sum  Inputs=++++  OutDataType=sfix(16)  OutScaling=2^0  SaturateOnIntegerOverflow=on  InputSameDT=on  OutDataTypeStr=Inherit: Same as first input
  CA_CO2 CA_O2 : Mux  Inputs=2
  CO2_A : Integrator  InitialCondition=m_CO2_alv_alvds_i
  Demux : Demux  Outputs=2
  Mux N2O O2 CO2 : Mux
  N2O,O2 CO2,N2 : Demux
  N2O_A : Integrator  InitialCondition=m_N2O_alv_alvds_i
  N2_A : Integrator  InitialCondition=m_N2_alv_alvds_i
  Net inflow CO2 : Sum  Inputs=+--  OutDataType=sfix(16)  OutScaling=2^0  SaturateOnIntegerOverflow=on  InputSameDT=on  OutDataTypeStr=Inherit: Same as first input
  Net inflow N2O : Sum  Inputs=-+  OutDataType=sfix(16)  OutScaling=2^0  SaturateOnIntegerOverflow=on  InputSameDT=on  OutDataTypeStr=Inherit: Same as first input
  Net inflow O2 : Sum  Inputs=-+-  OutDataType=sfix(16)  OutScaling=2^0  SaturateOnIntegerOverflow=on  InputSameDT=on  OutDataTypeStr=Inherit: Same as first input
  O2_A : Integrator  InitialCondition=m_O2_alv_alvds_i
  P{5..6,10..11} (4 alike) : Product  OutDataType=sfix(16)  OutScaling=2^0  SaturateOnIntegerOverflow=on  RndMeth=Zero  InputSameDT=on  OutDataTypeStr=Inherit: Same as first input
  P2 : Product  Inputs=*/  OutDataType=sfix(16)  OutScaling=2^0  SaturateOnIntegerOverflow=on  RndMeth=Zero  InputSameDT=on  OutDataTypeStr=Inherit: Same as first input
  P3 : Product  Inputs=/*  OutDataType=sfix(16)  OutScaling=2^0  SaturateOnIntegerOverflow=on  RndMeth=Zero  InputSameDT=on  OutDataTypeStr=Inherit: Same as first input
  P8 : Product  Inputs=/*  OutDataType=sfix(16)  OutScaling=2^0  SaturateOnIntegerOverflow=on  RndMeth=Zero  InputSameDT=on  OutDataTypeStr=Inherit: Same as first input
  P9 : Product  Inputs=/*  OutDataType=sfix(16)  OutScaling=2^0  SaturateOnIntegerOverflow=on  RndMeth=Zero  InputSameDT=on  OutDataTypeStr=Inherit: Same as first input
  To WS1 : ToWorkspace  VariableName=F_A_alvds_CO2  SampleTime=t_sample  SaveFormat=Array
  To WS2 : ToWorkspace  VariableName=F_A_alvds_O2  SampleTime=t_sample  SaveFormat=Array
  To WS3 : ToWorkspace  VariableName=m_alv_alvds  SampleTime=t_sample  SaveFormat=Array
  inflow N2 : Sum  Inputs=+-  OutDataType=sfix(16)  OutScaling=2^0  SaturateOnIntegerOverflow=on  InputSameDT=on  OutDataTypeStr=Inherit: Same as first input
  Exp flow  Out: : Outport  OutDataType=sfix(16)  OutScaling=2^0
  FA_gases : Outport  Port=2  OutDataType=sfix(16)  OutScaling=2^0
  tag scope: m_alv_alvds=global
  wires:
  N2O,O2 CO2,N2/1 -> Net inflow N2O/2
  Net inflow N2O/1 -> N2O_A/1
  Net inflow O2/1 -> O2_A/1
  Insp flow in/1 -> N2O,O2 CO2,N2/1
  Net inflow CO2/1 -> CO2_A/1
  N2O,O2 CO2,N2/2 -> Net inflow O2/2
  P6/1 -> Mux N2O O2 CO2/2, Net inflow O2/3
  P10/1 -> Mux N2O O2 CO2/3, Net inflow CO2/3
  N2O,O2 CO2,N2/3 -> Net inflow CO2/1
  Demux/1 -> Net inflow CO2/2
  Demux/2 -> Net inflow O2/1
  mdot_gases/1 -> Demux/1
  N2O,O2 CO2,N2/4 -> inflow N2/1
  P11/1 -> Mux N2O O2 CO2/4, inflow N2/2
  inflow N2/1 -> N2_A/1
  P5/1 -> Net inflow N2O/1, Mux N2O O2 CO2/1
  Alv vol/1 -> P9/1, P8/1, P3/1, P2/2, To WS3/1, [m_alv_alvds]
  Mux N2O O2 CO2/1 -> Exp flow  Out:/1
  O2_A/1 -> P3/2, Alv vol/2
  CA_CO2 CA_O2/1 -> FA_gases/1
  P8/1 -> P10/2, To WS1/1, CA_CO2 CA_O2/1
  P3/1 -> P6/2, To WS2/1, CA_CO2 CA_O2/2
  P2/1 -> P5/2
  CO2_A/1 -> Alv vol/3, P8/2
  N2O_A/1 -> Alv vol/1, P2/1
  N2_A/1 -> Alv vol/4, P9/2
  P9/1 -> P11/2
  [mdot_exp_alv_alvds] -> P11/1, P10/1, P6/1, P5/1

== system Resp18e_updatedPulse/Patient/Airways + alveoli/Alv compartment hi V/Q ==
  note: +ve out of alv
  note: molar conc
      | per unit
  Insp flow in : Inport  PortDimensions=4  OutDataType=sfix(16)  OutScaling=2^0
  mdot_gases : Inport  Port=2  PortDimensions=2  OutDataType=sfix(16)  OutScaling=2^0
  Alv vol : Sum  Inputs=++++  OutDataType=sfix(16)  OutScaling=2^0  SaturateOnIntegerOverflow=on  InputSameDT=on  OutDataTypeStr=Inherit: Same as first input
  CA_CO2 CA_O2 : Mux  Inputs=2
  CO2_A : Integrator  InitialCondition=m_CO2_alv_hivq_i
  Demux : Demux  Outputs=2
  Mux N2O O2 CO2 : Mux
  N2O,O2 CO2,N2 : Demux
  N2O_A : Integrator  InitialCondition=m_N2O_alv_hivq_i
  N2_A : Integrator  InitialCondition=m_N2_alv_hivq_i
  Net inflow CO2 : Sum  Inputs=+--  OutDataType=sfix(16)  OutScaling=2^0  SaturateOnIntegerOverflow=on  InputSameDT=on  OutDataTypeStr=Inherit: Same as first input
  Net inflow N2O : Sum  Inputs=-+  OutDataType=sfix(16)  OutScaling=2^0  SaturateOnIntegerOverflow=on  InputSameDT=on  OutDataTypeStr=Inherit: Same as first input
  Net inflow O2 : Sum  Inputs=-+-  OutDataType=sfix(16)  OutScaling=2^0  SaturateOnIntegerOverflow=on  InputSameDT=on  OutDataTypeStr=Inherit: Same as first input
  O2_A : Integrator  InitialCondition=m_O2_alv_hivq_i
  P{5..6,10..11} (4 alike) : Product  OutDataType=sfix(16)  OutScaling=2^0  SaturateOnIntegerOverflow=on  RndMeth=Zero  InputSameDT=on  OutDataTypeStr=Inherit: Same as first input
  P2 : Product  Inputs=*/  OutDataType=sfix(16)  OutScaling=2^0  SaturateOnIntegerOverflow=on  RndMeth=Zero  InputSameDT=on  OutDataTypeStr=Inherit: Same as first input
  P3 : Product  Inputs=/*  OutDataType=sfix(16)  OutScaling=2^0  SaturateOnIntegerOverflow=on  RndMeth=Zero  InputSameDT=on  OutDataTypeStr=Inherit: Same as first input
  P8 : Product  Inputs=/*  OutDataType=sfix(16)  OutScaling=2^0  SaturateOnIntegerOverflow=on  RndMeth=Zero  InputSameDT=on  OutDataTypeStr=Inherit: Same as first input
  P9 : Product  Inputs=/*  OutDataType=sfix(16)  OutScaling=2^0  SaturateOnIntegerOverflow=on  RndMeth=Zero  InputSameDT=on  OutDataTypeStr=Inherit: Same as first input
  To WS1 : ToWorkspace  VariableName=F_A_hivq_CO2  SampleTime=t_sample  SaveFormat=Array
  To WS2 : ToWorkspace  VariableName=F_A_hivq_O2  SampleTime=t_sample  SaveFormat=Array
  To WS3 : ToWorkspace  VariableName=m_alv_hivq  SampleTime=t_sample  SaveFormat=Array
  inflow N2 : Sum  Inputs=+-  OutDataType=sfix(16)  OutScaling=2^0  SaturateOnIntegerOverflow=on  InputSameDT=on  OutDataTypeStr=Inherit: Same as first input
  Exp flow  Out: : Outport  OutDataType=sfix(16)  OutScaling=2^0
  FA_gases : Outport  Port=2  OutDataType=sfix(16)  OutScaling=2^0
  tag scope: m_alv_hivq=global
  wires:
  P9/1 -> P11/2
  N2_A/1 -> P9/2, Alv vol/4
  N2O_A/1 -> P2/1, Alv vol/1
  CO2_A/1 -> P8/2, Alv vol/3
  P2/1 -> P5/2
  P3/1 -> CA_CO2 CA_O2/2, To WS2/1, P6/2
  P8/1 -> CA_CO2 CA_O2/1, To WS1/1, P10/2
  CA_CO2 CA_O2/1 -> FA_gases/1
  O2_A/1 -> Alv vol/2, P3/2
  Mux N2O O2 CO2/1 -> Exp flow  Out:/1
  Alv vol/1 -> P2/2, P3/1, P8/1, P9/1, [m_alv_hivq], To WS3/1
  P5/1 -> Mux N2O O2 CO2/1, Net inflow N2O/1
  inflow N2/1 -> N2_A/1
  P11/1 -> inflow N2/2, Mux N2O O2 CO2/4
  N2O,O2 CO2,N2/4 -> inflow N2/1
  mdot_gases/1 -> Demux/1
  Demux/2 -> Net inflow O2/1
  Demux/1 -> Net inflow CO2/2
  N2O,O2 CO2,N2/3 -> Net inflow CO2/1
  P10/1 -> Net inflow CO2/3, Mux N2O O2 CO2/3
  P6/1 -> Net inflow O2/3, Mux N2O O2 CO2/2
  N2O,O2 CO2,N2/2 -> Net inflow O2/2
  Net inflow CO2/1 -> CO2_A/1
  Insp flow in/1 -> N2O,O2 CO2,N2/1
  Net inflow O2/1 -> O2_A/1
  Net inflow N2O/1 -> N2O_A/1
  N2O,O2 CO2,N2/1 -> Net inflow N2O/2
  [mdot_exp_alv_hivq] -> P5/1, P6/1, P10/1, P11/1

== system Resp18e_updatedPulse/Patient/Airways + alveoli/Alv compartment lo V/Q ==
  note: +ve out of alv
  note: molar conc
      | per unit
  Insp flow in : Inport  PortDimensions=4  OutDataType=sfix(16)  OutScaling=2^0
  mdot_gases : Inport  Port=2  PortDimensions=2  OutDataType=sfix(16)  OutScaling=2^0
  Alv vol : Sum  Inputs=++++  OutDataType=sfix(16)  OutScaling=2^0  SaturateOnIntegerOverflow=on  InputSameDT=on  OutDataTypeStr=Inherit: Same as first input
  CA_CO2 CA_O2 : Mux  Inputs=2
  CO2_A : Integrator  InitialCondition=m_CO2_alv_lovq_i
  Demux : Demux  Outputs=2
  Mux N2O O2 CO2 : Mux
  N2O,O2 CO2,N2 : Demux
  N2O_A : Integrator  InitialCondition=m_N2O_alv_lovq_i
  N2_A : Integrator  InitialCondition=m_N2_alv_lovq_i
  Net inflow CO2 : Sum  Inputs=+--  OutDataType=sfix(16)  OutScaling=2^0  SaturateOnIntegerOverflow=on  InputSameDT=on  OutDataTypeStr=Inherit: Same as first input
  Net inflow N2O : Sum  Inputs=-+  OutDataType=sfix(16)  OutScaling=2^0  SaturateOnIntegerOverflow=on  InputSameDT=on  OutDataTypeStr=Inherit: Same as first input
  Net inflow O2 : Sum  Inputs=-+-  OutDataType=sfix(16)  OutScaling=2^0  SaturateOnIntegerOverflow=on  InputSameDT=on  OutDataTypeStr=Inherit: Same as first input
  O2_A : Integrator  InitialCondition=m_O2_alv_lovq_i
  P{5..6,10..11} (4 alike) : Product  OutDataType=sfix(16)  OutScaling=2^0  SaturateOnIntegerOverflow=on  RndMeth=Zero  InputSameDT=on  OutDataTypeStr=Inherit: Same as first input
  P2 : Product  Inputs=*/  OutDataType=sfix(16)  OutScaling=2^0  SaturateOnIntegerOverflow=on  RndMeth=Zero  InputSameDT=on  OutDataTypeStr=Inherit: Same as first input
  P3 : Product  Inputs=/*  OutDataType=sfix(16)  OutScaling=2^0  SaturateOnIntegerOverflow=on  RndMeth=Zero  InputSameDT=on  OutDataTypeStr=Inherit: Same as first input
  P8 : Product  Inputs=/*  OutDataType=sfix(16)  OutScaling=2^0  SaturateOnIntegerOverflow=on  RndMeth=Zero  InputSameDT=on  OutDataTypeStr=Inherit: Same as first input
  P9 : Product  Inputs=/*  OutDataType=sfix(16)  OutScaling=2^0  SaturateOnIntegerOverflow=on  RndMeth=Zero  InputSameDT=on  OutDataTypeStr=Inherit: Same as first input
  To WS1 : ToWorkspace  VariableName=F_A_lovq_CO2  SampleTime=t_sample  SaveFormat=Array
  To WS2 : ToWorkspace  VariableName=F_A_lovq_O2  SampleTime=t_sample  SaveFormat=Array
  To WS3 : ToWorkspace  VariableName=m_alv_lovq  SampleTime=t_sample  SaveFormat=Array
  inflow N2 : Sum  Inputs=+-  OutDataType=sfix(16)  OutScaling=2^0  SaturateOnIntegerOverflow=on  InputSameDT=on  OutDataTypeStr=Inherit: Same as first input
  Exp flow  Out: : Outport  OutDataType=sfix(16)  OutScaling=2^0
  FA_gases : Outport  Port=2  OutDataType=sfix(16)  OutScaling=2^0
  tag scope: m_alv_lovq=global
  wires:
  P9/1 -> P11/2
  N2_A/1 -> P9/2, Alv vol/4
  N2O_A/1 -> P2/1, Alv vol/1
  CO2_A/1 -> P8/2, Alv vol/3
  P2/1 -> P5/2
  P3/1 -> CA_CO2 CA_O2/2, To WS2/1, P6/2
  P8/1 -> CA_CO2 CA_O2/1, To WS1/1, P10/2
  CA_CO2 CA_O2/1 -> FA_gases/1
  O2_A/1 -> Alv vol/2, P3/2
  Mux N2O O2 CO2/1 -> Exp flow  Out:/1
  Alv vol/1 -> P2/2, P3/1, P8/1, P9/1, [m_alv_lovq], To WS3/1
  P5/1 -> Mux N2O O2 CO2/1, Net inflow N2O/1
  inflow N2/1 -> N2_A/1
  P11/1 -> inflow N2/2, Mux N2O O2 CO2/4
  N2O,O2 CO2,N2/4 -> inflow N2/1
  mdot_gases/1 -> Demux/1
  Demux/2 -> Net inflow O2/1
  Demux/1 -> Net inflow CO2/2
  N2O,O2 CO2,N2/3 -> Net inflow CO2/1
  P10/1 -> Net inflow CO2/3, Mux N2O O2 CO2/3
  P6/1 -> Net inflow O2/3, Mux N2O O2 CO2/2
  N2O,O2 CO2,N2/2 -> Net inflow O2/2
  Net inflow CO2/1 -> CO2_A/1
  Insp flow in/1 -> N2O,O2 CO2,N2/1
  Net inflow O2/1 -> O2_A/1
  Net inflow N2O/1 -> N2O_A/1
  N2O,O2 CO2,N2/1 -> Net inflow N2O/2
  [mdot_exp_alv_lovq] -> P5/1, P6/1, P10/1, P11/1

== system Resp18e_updatedPulse/Patient/Airways + alveoli/Alv compartment mid V/Q ==
  note: molar conc
      | per unit
  note: +ve out of alv
  Insp flow in : Inport  PortDimensions=4  OutDataType=sfix(16)  OutScaling=2^0
  mdot_gases : Inport  Port=2  PortDimensions=2  OutDataType=sfix(16)  OutScaling=2^0
  Alv vol : Sum  Inputs=++++  OutDataType=sfix(16)  OutScaling=2^0  SaturateOnIntegerOverflow=on  InputSameDT=on  OutDataTypeStr=Inherit: Same as first input
  CA_CO2 CA_O2 : Mux  Inputs=2
  CO2_A : Integrator  InitialCondition=m_CO2_alv_midvq_i
  Demux : Demux  Outputs=2
  Mux N2O O2 CO2 : Mux
  N2O,O2 CO2,N2 : Demux
  N2O_A : Integrator  InitialCondition=m_N2O_alv_midvq_i
  N2_A : Integrator  InitialCondition=m_N2_alv_midvq_i
  Net inflow CO2 : Sum  Inputs=+--  OutDataType=sfix(16)  OutScaling=2^0  SaturateOnIntegerOverflow=on  InputSameDT=on  OutDataTypeStr=Inherit: Same as first input
  Net inflow N2O : Sum  Inputs=-+  OutDataType=sfix(16)  OutScaling=2^0  SaturateOnIntegerOverflow=on  InputSameDT=on  OutDataTypeStr=Inherit: Same as first input
  Net inflow O2 : Sum  Inputs=-+-  OutDataType=sfix(16)  OutScaling=2^0  SaturateOnIntegerOverflow=on  InputSameDT=on  OutDataTypeStr=Inherit: Same as first input
  O2_A : Integrator  InitialCondition=m_O2_alv_midvq_i
  P{5..6,10..11} (4 alike) : Product  OutDataType=sfix(16)  OutScaling=2^0  SaturateOnIntegerOverflow=on  RndMeth=Zero  InputSameDT=on  OutDataTypeStr=Inherit: Same as first input
  P2 : Product  Inputs=*/  OutDataType=sfix(16)  OutScaling=2^0  SaturateOnIntegerOverflow=on  RndMeth=Zero  InputSameDT=on  OutDataTypeStr=Inherit: Same as first input
  P3 : Product  Inputs=/*  OutDataType=sfix(16)  OutScaling=2^0  SaturateOnIntegerOverflow=on  RndMeth=Zero  InputSameDT=on  OutDataTypeStr=Inherit: Same as first input
  P8 : Product  Inputs=/*  OutDataType=sfix(16)  OutScaling=2^0  SaturateOnIntegerOverflow=on  RndMeth=Zero  InputSameDT=on  OutDataTypeStr=Inherit: Same as first input
  P9 : Product  Inputs=/*  OutDataType=sfix(16)  OutScaling=2^0  SaturateOnIntegerOverflow=on  RndMeth=Zero  InputSameDT=on  OutDataTypeStr=Inherit: Same as first input
  To WS1 : ToWorkspace  VariableName=F_A_midvq_CO2  SampleTime=t_sample  SaveFormat=Array
  To WS2 : ToWorkspace  VariableName=F_A_midvq_O2  SampleTime=t_sample  SaveFormat=Array
  To WS3 : ToWorkspace  VariableName=m_alv_midvq  SampleTime=t_sample  SaveFormat=Array
  inflow N2 : Sum  Inputs=+-  OutDataType=sfix(16)  OutScaling=2^0  SaturateOnIntegerOverflow=on  InputSameDT=on  OutDataTypeStr=Inherit: Same as first input
  Exp flow  Out: : Outport  OutDataType=sfix(16)  OutScaling=2^0
  FA_gases : Outport  Port=2  OutDataType=sfix(16)  OutScaling=2^0
  tag scope: m_alv_midvq=global
  wires:
  N2O,O2 CO2,N2/1 -> Net inflow N2O/2
  Net inflow N2O/1 -> N2O_A/1
  Net inflow O2/1 -> O2_A/1
  Insp flow in/1 -> N2O,O2 CO2,N2/1
  Net inflow CO2/1 -> CO2_A/1
  N2O,O2 CO2,N2/2 -> Net inflow O2/2
  P6/1 -> Mux N2O O2 CO2/2, Net inflow O2/3
  P10/1 -> Mux N2O O2 CO2/3, Net inflow CO2/3
  N2O,O2 CO2,N2/3 -> Net inflow CO2/1
  Demux/1 -> Net inflow CO2/2
  Demux/2 -> Net inflow O2/1
  mdot_gases/1 -> Demux/1
  N2O,O2 CO2,N2/4 -> inflow N2/1
  P11/1 -> Mux N2O O2 CO2/4, inflow N2/2
  inflow N2/1 -> N2_A/1
  P5/1 -> Net inflow N2O/1, Mux N2O O2 CO2/1
  Alv vol/1 -> P9/1, P8/1, P3/1, P2/2, [m_alv_midvq], To WS3/1
  Mux N2O O2 CO2/1 -> Exp flow  Out:/1
  O2_A/1 -> P3/2, Alv vol/2
  CA_CO2 CA_O2/1 -> FA_gases/1
  P8/1 -> P10/2, To WS1/1, CA_CO2 CA_O2/1
  P3/1 -> P6/2, To WS2/1, CA_CO2 CA_O2/2
  P2/1 -> P5/2
  CO2_A/1 -> Alv vol/3, P8/2
  N2O_A/1 -> Alv vol/1, P2/1
  N2_A/1 -> Alv vol/4, P9/2
  P9/1 -> P11/2
  [mdot_exp_alv_midvq] -> P11/1, P10/1, P6/1, P5/1
